simulink model "OBJMIL"  (Simulink 8.2)
settings: Solver=FixedStepDiscrete  StartTime=0.0  StopTime=126  FixedStep=0.005  RelTol=1e-3
PostLoadFcn:
  | , if any(exist('dsrtsu_mdlpostloadfcn', 'file') == [2, 3, 6]), try dsrtsu_mdlpostloadfcn('Execute', bdroot); catch fprintf('Error in PostLoadFcn (dsrtsu_mdlpostloadfcn) for model "%s":\n %s\n', bdroot, lasterr); end, end,
values from neighbouring files (symbols this model uses):
  C_TASK_5MS_S = (	C_TICK_TIME_S      	)    [hcu_local_hdr.m]
  ENUM_GEARPOSN_1ST = uint8(  1  )    [hcu_local_hdr.m]
  ENUM_GEARPOSN_R = uint8(  7  )    [hcu_local_hdr.m]
  FALSE = boolean( 0 )    [hcu_local_hdr.m]
  R_OBJ_Position = single([ii 0 0])    [GridSearch.m]
  R_OBJ_RelAccel = single([0 0 kk])    [GridSearch.m]
  R_OBJ_RelVelocity = single([0 jj 0])    [GridSearch.m]
  TRUE = boolean( 1 )    [hcu_local_hdr.m]
undefined symbols (not defined in the file or in its folder): A_OBJ, B_OBJ, C_OBJ, Gamma_OBJ, KOBJ_KalmanFilterCalRate_s, KOBJ_UseCalObjSpd_flg, KOBJ_UseEstObjInfo_flg, KOBJ_VehAccCalRate_s, KOBJ_VehAccFltConst_s, Q_OBJ, slcm
libraries: simulink x39, hcu_lib x10, dspmtrx3 x3, dspinverses x1
(part 2 of 2)

== system OBJMIL/OBJ/OBJ/Obj4_RelVelocity_Calculation/Obj4_RelVelocity_Cal ==
  ObjPositionX_m : Inport
  TimeDur_s : Inport  Port=2
  Trigger : TriggerPort
  Compare To Zero1 : simulink/Logic and Bit Operations/Compare To Zero  relop=~=  OutDataTypeStr=boolean
  Compare To Zero2 : simulink/Logic and Bit Operations/Compare To Zero  relop=~=  OutDataTypeStr=boolean
  Compare To Zero3 : simulink/Logic and Bit Operations/Compare To Zero  relop=~=  OutDataTypeStr=boolean
  Constant1 : Constant  Value=0  OutDataTypeStr=single
  Enabled Subsystem : Subsystem  TreatAsAtomicUnit=on
  Logical Operator : Logic  Inputs=3  AllPortsSameDT=off  OutDataTypeStr=boolean
  Sum : Sum  Inputs=+-
  Unit Delay : UnitDelay  SampleTime=-1
  Unit Delay2 : UnitDelay  SampleTime=-1
  divide : hcu_lib/divide
  VOBJ_Obj4RelVelocityCal_mps : Outport
  wires:
  divide/1 -> VOBJ_Obj4RelVelocityCal_mps/1  "VOBJ_Obj4RelVelocityCal_mps"
  Unit Delay/1 -> Compare To Zero2/1, Unit Delay2/1, Sum/2
  ObjPositionX_m/1 -> Compare To Zero1/1, Sum/1, Unit Delay/1
  TimeDur_s/1 -> divide/2
  Constant1/1 -> divide/3
  Compare To Zero1/1 -> Logical Operator/1
  Compare To Zero2/1 -> Logical Operator/2
  Logical Operator/1 -> Enabled Subsystem/Enable
  Sum/1 -> Enabled Subsystem/1(In1)
  Enabled Subsystem/1(Out1) -> divide/1
  Compare To Zero3/1 -> Logical Operator/3
  Unit Delay2/1 -> Compare To Zero3/1

== system OBJMIL/OBJ/OBJ/Obj4_RelVelocity_Calculation/SandH_Obj4 ==
  In1 : Inport
  Trigger : TriggerPort
  Out1 : Outport
  wires:
  In1/1 -> Out1/1

== system OBJMIL/OBJ/OBJ/Obj4_RelVelocity_Calculation/Timer4 ==
  Enable : EnablePort  StatesWhenEnabling=reset  ZeroCross=off
  Constant : Constant  Value=C_TASK_5MS_S
  Sum : Sum  Inputs=|++  SaturateOnIntegerOverflow=on  InputSameDT=on
  Unit Delay : UnitDelay  SampleTime=-1
  Timer (sec) : Outport  OutputWhenDisabled=reset  InitialOutput=0
  wires:
  Unit Delay/1 -> Timer (sec)/1, Sum/2
  Sum/1 -> Unit Delay/1
  Constant/1 -> Sum/1

== system OBJMIL/OBJ/OBJ/Obj5_RelVelocity_Calculation/DataPass_Obj5 ==
  In1 : Inport
  Enable : EnablePort  StatesWhenEnabling=reset
  Out1 : Outport  OutputWhenDisabled=reset  InitialOutput=[0]
  wires:
  In1/1 -> Out1/1

== system OBJMIL/OBJ/OBJ/Obj5_RelVelocity_Calculation/Obj5_RelVelocity_Cal ==
  ObjPositionX_m : Inport
  TimeDur_s : Inport  Port=2
  Trigger : TriggerPort
  Compare To Zero1 : simulink/Logic and Bit Operations/Compare To Zero  relop=~=  OutDataTypeStr=boolean
  Compare To Zero2 : simulink/Logic and Bit Operations/Compare To Zero  relop=~=  OutDataTypeStr=boolean
  Compare To Zero3 : simulink/Logic and Bit Operations/Compare To Zero  relop=~=  OutDataTypeStr=boolean
  Constant1 : Constant  Value=0  OutDataTypeStr=single
  Enabled Subsystem : Subsystem  TreatAsAtomicUnit=on
  Logical Operator : Logic  Inputs=3  AllPortsSameDT=off  OutDataTypeStr=boolean
  Sum : Sum  Inputs=+-
  Unit Delay : UnitDelay  SampleTime=-1
  Unit Delay2 : UnitDelay  SampleTime=-1
  divide : hcu_lib/divide
  VOBJ_Obj5RelVelocityCal_mps : Outport
  wires:
  Unit Delay2/1 -> Compare To Zero3/1
  Compare To Zero3/1 -> Logical Operator/3
  Enabled Subsystem/1(Out1) -> divide/1
  Sum/1 -> Enabled Subsystem/1(In1)
  Logical Operator/1 -> Enabled Subsystem/Enable
  Compare To Zero2/1 -> Logical Operator/2
  Compare To Zero1/1 -> Logical Operator/1
  Constant1/1 -> divide/3
  TimeDur_s/1 -> divide/2
  ObjPositionX_m/1 -> Unit Delay/1, Sum/1, Compare To Zero1/1
  Unit Delay/1 -> Sum/2, Unit Delay2/1, Compare To Zero2/1
  divide/1 -> VOBJ_Obj5RelVelocityCal_mps/1  "VOBJ_Obj5RelVelocityCal_mps"

== system OBJMIL/OBJ/OBJ/Obj5_RelVelocity_Calculation/SandH_Obj5 ==
  In1 : Inport
  Trigger : TriggerPort
  Out1 : Outport
  wires:
  In1/1 -> Out1/1

== system OBJMIL/OBJ/OBJ/Obj5_RelVelocity_Calculation/Timer5 ==
  Enable : EnablePort  StatesWhenEnabling=reset  ZeroCross=off
  Constant : Constant  Value=C_TASK_5MS_S
  Sum : Sum  Inputs=|++  SaturateOnIntegerOverflow=on  InputSameDT=on
  Unit Delay : UnitDelay  SampleTime=-1
  Timer (sec) : Outport  OutputWhenDisabled=reset  InitialOutput=0
  wires:
  Constant/1 -> Sum/1
  Sum/1 -> Unit Delay/1
  Unit Delay/1 -> Sum/2, Timer (sec)/1

== system OBJMIL/OBJ/OBJ/Trigger signal generator/trigger signal generator ==
  Time_dur [s] : Inport
  Constant3 : Constant  Value=0  OutDataTypeStr=single
  Constant4 : Constant  Value=C_TASK_5MS_S
  Relational Operator1 : RelationalOperator  OutDataTypeStr=boolean
  Sum1 : Sum  Inputs=|++  SaturateOnIntegerOverflow=on  InputSameDT=on
  Sum2 : Sum  Inputs=+-
  Switch3 : Switch  Threshold=0.5
  Unit Delay2 : UnitDelay  SampleTime=-1
  Unit Delay3 : UnitDelay  SampleTime=-1
  Trigger_signal : Outport  OutputWhenDisabled=reset  InitialOutput=[0]
  wires:
  Sum2/1 -> Relational Operator1/2
  Unit Delay3/1 -> Switch3/2
  Unit Delay2/1 -> Sum1/2
  Switch3/1 -> Relational Operator1/1, Unit Delay2/1
  Constant3/1 -> Switch3/1
  Time_dur [s]/1 -> Sum2/1
  Relational Operator1/1 -> Unit Delay3/1, Trigger_signal/1
  Constant4/1 -> Sum2/2, Sum1/1
  Sum1/1 -> Switch3/3

== system OBJMIL/OBJ/OBJ/Trigger signal generator1/trigger signal generator ==
  Time_dur [s] : Inport
  Constant3 : Constant  Value=0  OutDataTypeStr=single
  Constant4 : Constant  Value=C_TASK_5MS_S
  Relational Operator1 : RelationalOperator  OutDataTypeStr=boolean
  Sum1 : Sum  Inputs=|++  SaturateOnIntegerOverflow=on  InputSameDT=on
  Sum2 : Sum  Inputs=+-
  Switch3 : Switch  Threshold=0.5
  Unit Delay2 : UnitDelay  SampleTime=-1
  Unit Delay3 : UnitDelay  SampleTime=-1
  Trigger_signal : Outport  OutputWhenDisabled=reset  InitialOutput=[0]
  wires:
  Sum2/1 -> Relational Operator1/2
  Unit Delay3/1 -> Switch3/2
  Unit Delay2/1 -> Sum1/2
  Switch3/1 -> Relational Operator1/1, Unit Delay2/1
  Constant3/1 -> Switch3/1
  Time_dur [s]/1 -> Sum2/1
  Relational Operator1/1 -> Unit Delay3/1, Trigger_signal/1
  Constant4/1 -> Sum2/2, Sum1/1
  Sum1/1 -> Switch3/3

== system OBJMIL/OBJ/OBJ/Vehicle Acceleration Calculation/signal_filter ==
  raw_input : Inport
  Tc : Inport  Port=2
  Ts : Inport  Port=3
  FirstOrderFilter : Subsystem  RTWFileName=HCU_LIB
      settings: RTWFileNameOpts=User specified
  IC : UnitDelay  Tag=struct('comment',struct('text','','placement',1),'logdata',struct('maxnumvals',inf,'plotchannels',[],'stepsize',0,'downsampling',1,'loggingmode',3,'channels',1),'output',struct('width',1,'name','$S_$B','unit','','type','Int16','offset',0,'max',NaN,'min',NaN,'freeze',1,'lsb',1,'arb',0,'class','default','address','','description','','autoscalingmode',1,'lowerheadroom',1,'upperheadroom',1,'headroomunit','bit','checkmin',0,'checkmax',0,'show',0,'initial','2'),'state',0,'dt','-1','date',731455.586925799)  SampleTime=-1
  Switch1 : Switch  Tag=struct('comment',struct('text','','placement',1),'logdata',struct('maxnumvals',inf,'plotchannels',[],'stepsize',0,'downsampling',1,'loggingmode',3,'channels',1),'output',struct('width',1,'name','$S_$B','unit','','type','Int32Bin15','offset',0,'max',65535,'min',-65536,'freeze',1,'lsb',2^-15,'arb',0,'class','default','address','','description','','autoscalingmode',1,'lowerheadroom',1,'upperheadroom',1,'headroomunit','bit','checkmin',0,'checkmax',0,'show',0),'threshold',struct('width',1,'name','$S_$B_threshold','unit','','type','Int16','offset',0,'max',NaN,'min',NaN,'freeze',1,'lsb',1,'arb',0,'class','default','address','','description','','value','1','scalar',0),'date',731455.58657044)  Threshold=0.5  InputSameDT=on
  zero : Constant  Tag=struct('comment',struct('text','','placement',1),'output',struct('width',1,'name','$S_$B','unit','','type','Int16','offset',0,'max',NaN,'min',NaN,'freeze',1,'lsb',1,'arb',0,'class','default','address','','description','','value','0','tolerance',1,'show',0),'date',731455.58675544)  Value=TRUE
  zero1 : Constant  Tag=struct('comment',struct('text','','placement',1),'output',struct('width',1,'name','$S_$B','unit','','type','Int16','offset',0,'max',NaN,'min',NaN,'freeze',1,'lsb',1,'arb',0,'class','default','address','','description','','value','0','tolerance',1,'show',0),'date',731455.58675544)  Value=0  OutDataTypeStr=single
  raw_input_filt : Outport
  wires:
  zero/1 -> IC/1
  raw_input/1 -> FirstOrderFilter/1(in)
  Tc/1 -> Switch1/1
  Ts/1 -> FirstOrderFilter/3(Ts)
  IC/1 -> Switch1/2
  FirstOrderFilter/1(out) -> raw_input_filt/1
  Switch1/1 -> FirstOrderFilter/2(Tc)
  zero1/1 -> Switch1/3

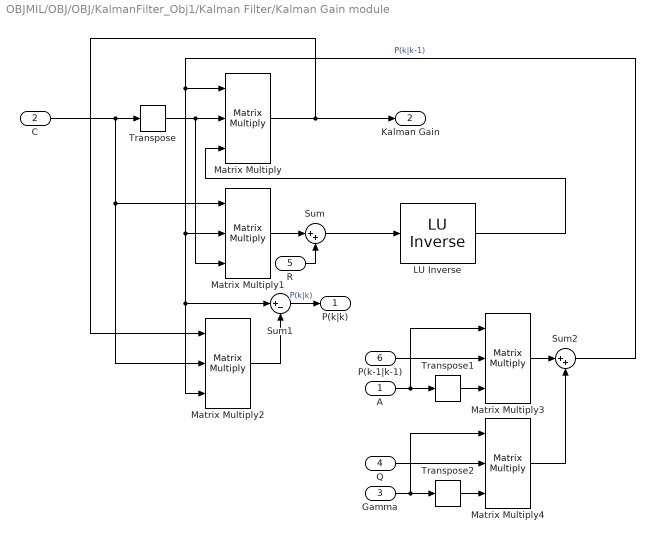
== system OBJMIL/OBJ/OBJ/KalmanFilter_Obj1/Kalman Filter/Kalman Gain module ==
  A : Inport
  C : Inport  Port=2
  Gamma : Inport  Port=3
  Q : Inport  Port=4
  R : Inport  Port=5
  P(k-1|k-1) : Inport  Port=6
  " LU Inverse" : dspinverses/ LU Inverse
  Matrix Multiply{,1..4} (5 alike) : Product  Inputs=3  Multiplication=Matrix(*)
  Sum : Sum  Inputs=|++
  Sum1 : Sum  Inputs=|+-
  Sum2 : Sum  Inputs=|++
  Transpose : dspmtrx3/Transpose  Hermitian=off  overflowFlag=on
  Transpose1 : dspmtrx3/Transpose  Hermitian=off  overflowFlag=on
  Transpose2 : dspmtrx3/Transpose  Hermitian=off  overflowFlag=on
  P(k|k) : Outport
  Kalman Gain : Outport  Port=2
  wires:
  C/1 -> Transpose/1, Matrix Multiply1/1, Matrix Multiply2/2
  Transpose/1 -> Matrix Multiply/2, Matrix Multiply1/3
  Matrix Multiply1/1 -> Sum/1
  R/1 -> Sum/2
  Sum/1 -> " LU Inverse"/1
  " LU Inverse"/1 -> Matrix Multiply/3
  Matrix Multiply/1 -> Matrix Multiply2/1, Kalman Gain/1
  Matrix Multiply2/1 -> Sum1/2
  A/1 -> Transpose1/1, Matrix Multiply3/1
  Transpose1/1 -> Matrix Multiply3/3
  Matrix Multiply3/1 -> Sum2/1
  Transpose2/1 -> Matrix Multiply4/3
  Gamma/1 -> Transpose2/1, Matrix Multiply4/1
  Q/1 -> Matrix Multiply4/2
  Matrix Multiply4/1 -> Sum2/2
  Sum2/1 -> Matrix Multiply/1, Matrix Multiply1/2, Sum1/1, Matrix Multiply2/3  "P(k|k-1)"
  P(k-1|k-1)/1 -> Matrix Multiply3/2
  Sum1/1 -> P(k|k)/1  "P(k|k)"

== system OBJMIL/OBJ/OBJ/Obj1_RelVelocity_Calculation/Obj1_RelVelocity_Cal/Enabled Subsystem ==
  In1 : Inport
  Enable : EnablePort  StatesWhenEnabling=reset
  Out1 : Outport  OutputWhenDisabled=reset  InitialOutput=[0]
  wires:
  In1/1 -> Out1/1

== system OBJMIL/OBJ/OBJ/Obj2_RelVelocity_Calculation/Obj2_RelVelocity_Cal/Enabled Subsystem ==
  In1 : Inport
  Enable : EnablePort  StatesWhenEnabling=reset
  Out1 : Outport  OutputWhenDisabled=reset  InitialOutput=[0]
  wires:
  In1/1 -> Out1/1

== system OBJMIL/OBJ/OBJ/Obj3_RelVelocity_Calculation/Obj3_RelVelocity_Cal/Enabled Subsystem ==
  In1 : Inport
  Enable : EnablePort  StatesWhenEnabling=reset
  Out1 : Outport  OutputWhenDisabled=reset  InitialOutput=[0]
  wires:
  In1/1 -> Out1/1

== system OBJMIL/OBJ/OBJ/Obj4_RelVelocity_Calculation/Obj4_RelVelocity_Cal/Enabled Subsystem ==
  In1 : Inport
  Enable : EnablePort  StatesWhenEnabling=reset
  Out1 : Outport  OutputWhenDisabled=reset  InitialOutput=[0]
  wires:
  In1/1 -> Out1/1

== system OBJMIL/OBJ/OBJ/Obj5_RelVelocity_Calculation/Obj5_RelVelocity_Cal/Enabled Subsystem ==
  In1 : Inport
  Enable : EnablePort  StatesWhenEnabling=reset
  Out1 : Outport  OutputWhenDisabled=reset  InitialOutput=[0]
  wires:
  In1/1 -> Out1/1

== system OBJMIL/OBJ/OBJ/Vehicle Acceleration Calculation/signal_filter/FirstOrderFilter ==
  in : Inport
  Tc : Inport  Port=2
  Ts : Inport  Port=3
  Add : Sum
  Add1 : Sum
  Add2 : Sum  Inputs=+-
  Constant : Constant  OutDataTypeStr=single
  Divide : Product  Inputs=*/
  Product : Product  RndMeth=Zero
  Product1 : Product  RndMeth=Zero
  Unit Delay : UnitDelay  SampleTime=-1
  out : Outport
  wires:
  Add/1 -> Unit Delay/1, out/1
  Product1/1 -> Add/2
  Product/1 -> Add/1
  Add2/1 -> Product/2
  in/1 -> Product/1
  Divide/1 -> Product1/1, Add2/2
  Constant/1 -> Add2/1
  Add1/1 -> Divide/2
  Ts/1 -> Add1/2
  Tc/1 -> Divide/1, Add1/1
  Unit Delay/1 -> Product1/2

== stateflow chart Scheduler ==
  (default) -> (junction 10)
  (junction 10) -> (junction 11) : {
      | trig_DINR; ...
      | trig_TRCK; ...
      | trig_OBJ; ...
      | trig_PTH; ...
      | trig_MCT;...
      | trig_TTC; ...
      | trig_AEB; ...
      | }
  events: trig_DINR output FUNCTION_CALL_EVENT; trig_TRCK output FUNCTION_CALL_EVENT; trig_OBJ output FUNCTION_CALL_EVENT; trig_PTH output FUNCTION_CALL_EVENT; trig_MCT output FUNCTION_CALL_EVENT; trig_TTC output FUNCTION_CALL_EVENT; trig_AEB output FUNCTION_CALL_EVENT
